simulink model "Flatten1"  (Simulink 7.9)
settings: Solver=ode45  StartTime=0.0  StopTime=10.0  RelTol=1e-3
settings Model: Creator=boakes  LastModifiedBy=boakes

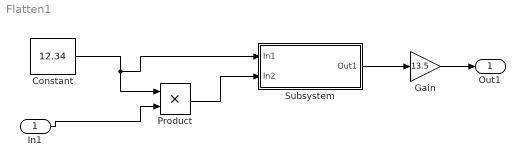
== system Flatten1 ==
  In1 : Inport
  Constant : Constant  Value=12.34
  Gain : Gain  Gain=13.5
  Product : Product  RndMeth=Zero
  Subsystem : Subsystem
  Out1 : Outport
  wires:
  Constant/1 -> Product/1, Subsystem/1(In1)
  In1/1 -> Product/2
  Product/1 -> Subsystem/2(In2)
  Subsystem/1(Out1) -> Gain/1
  Gain/1 -> Out1/1

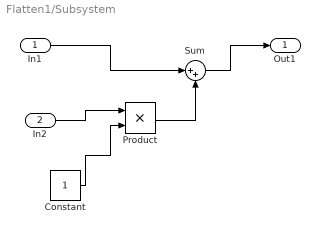
== system Flatten1/Subsystem ==
  In1 : Inport
  In2 : Inport  Port=2
  Constant : Constant
  Product : Product  RndMeth=Zero
  Sum : Sum  Inputs=|++
  Out1 : Outport
  wires:
  In2/1 -> Product/1
  Constant/1 -> Product/2
  In1/1 -> Sum/1
  Product/1 -> Sum/2
  Sum/1 -> Out1/1
